simulink model "BatteryStoragePVPlantGFM"  (R2023a)
settings: Solver=FixedStepDiscrete  StartTime=0.0  StopTime=SimulationTime  RelTol=1e-3
PreLoadFcn:
  | run('BatteryStoragePVPlantGFMParameters')
undefined symbols (not defined in the file): Array, Base, battery, BatteryInverter, DiscIntNeverNeededParam, ee, Feeder, fRT, GFLBatteryController, GFMBatteryController, Grid, GridTransformer, Line, Load, Load2CB_final, Load2CB_initial, LVRT, maxSoC, maxVdc, minIrrad, minSoC, minVdc, Mpp, olTime, Panel, PVController, PVInverter, PVTransformer, Scenario, SM, SubTransmissionLine, Ts, VSMbase
libraries: ee_lib x51, nesl_utility x45, fl_lib x26, eeGeneralControl x18, simulink x12, eeTransforms x11, slpidlib x8, eePowerMeasurement x5, batteryecm_lib x2, eeTotalHarmonicDistorsion x2, spsLeadLagFilterLib x1, eeSmAC1C x1
(part 2 of 5)

== system BatteryStoragePVPlantGFM/Transmission Line/CB ==
  Circuit Breaker Step off3 : ee_lib/Switches & Breakers/Circuit Breaker (Three-Phase)  R_closed=0.001 Ohm  G_open=1e-4 1/Ohm  threshold=0.5 V  breaker_behavior=ee.enum.switches.breakerBehavior.zeroCrossingEnable
      settings: InternalSimscapePortConfiguration="{\"Bottom\":[],\"Left\":[{\"id\":\"vT\",\"label\":\"vT\",\"type\":\"input\"},{\"id\":\"N1\",\"label\":\"~1\",\"type\":\"foundation.electrical.three_phase\"}],\"Right\":[{\"id\":\"N2\",\"label\":\"~2\",\"type\":\"foundation.electrical.three_phase\"}],\"Top\":[]}"
  Constant : Constant  Value=0
  Simulink-PS Converter3 : nesl_utility/Simulink-PS Converter  PhysicalDomain=network_engine_domain  SubClassName=ps_input  LeftPortType=input  RightPortType=output  PseudoPeriodic=off  Frequencies=[]  NoiseDistribution=none  NoiseParameters=[]  Unit=1  AffineConversion=off  FilteringAndDerivatives=zero  SimscapeFilterOrder=1  InputFilterTimeConstant=0.001  UdotUserProvided=1
  Conn1 : PMIOPort  Side=Right
  Conn2 : PMIOPort  Port=2  Side=Left
  wires:
  Constant/1 -> Simulink-PS Converter3/1
  connections:
  Circuit Breaker Step off3/LConn2 -- Conn2/RConn1
  Circuit Breaker Step off3/LConn1 -- Simulink-PS Converter3/RConn1
  Circuit Breaker Step off3/RConn1 -- Conn1/RConn1

== system BatteryStoragePVPlantGFM/Transmission Line/CB5 ==
  Circuit Breaker Step off3 : ee_lib/Switches & Breakers/Circuit Breaker (Three-Phase)  R_closed=0.001 Ohm  G_open=1e-4 1/Ohm  threshold=0.5 V  breaker_behavior=ee.enum.switches.breakerBehavior.zeroCrossingEnable
      settings: InternalSimscapePortConfiguration="{\"Bottom\":[],\"Left\":[{\"id\":\"vT\",\"label\":\"vT\",\"type\":\"input\"},{\"id\":\"N1\",\"label\":\"~1\",\"type\":\"foundation.electrical.three_phase\"}],\"Right\":[{\"id\":\"N2\",\"label\":\"~2\",\"type\":\"foundation.electrical.three_phase\"}],\"Top\":[]}"
  Constant : Constant  Value=0
  Simulink-PS Converter3 : nesl_utility/Simulink-PS Converter  PhysicalDomain=network_engine_domain  SubClassName=ps_input  LeftPortType=input  RightPortType=output  PseudoPeriodic=off  Frequencies=[]  NoiseDistribution=none  NoiseParameters=[]  Unit=1  AffineConversion=off  FilteringAndDerivatives=zero  SimscapeFilterOrder=1  InputFilterTimeConstant=0.001  UdotUserProvided=1
  Conn1 : PMIOPort  Side=Right
  Conn2 : PMIOPort  Port=2  Side=Left
  wires:
  Constant/1 -> Simulink-PS Converter3/1
  connections:
  Circuit Breaker Step off3/LConn2 -- Conn2/RConn1
  Circuit Breaker Step off3/LConn1 -- Simulink-PS Converter3/RConn1
  Circuit Breaker Step off3/RConn1 -- Conn1/RConn1

== system BatteryStoragePVPlantGFM/BESS & PV PARK/100 MWp PV Park/Measurement1 ==
  u : Inport
  Lead-Lag (Discrete or Continuous) : eeGeneralControl/Lead-Lag (Discrete or Continuous)  T1=0  T2=PVController.t_sensor  B=inf  A=-inf  init_option=Inherited from block input  x0=0  Ts=Ts
      settings: LibrarySourceBlock=|
      | ee_sl_lib/General Control/Lead-Lag
      | (Discrete or Continuous)
  Out Bus Element : Outport  PortName=ipv1  Element=1
  wires:
  Lead-Lag (Discrete or Continuous)/1 -> Out Bus Element/1
  u/1 -> Lead-Lag (Discrete or Continuous)/1

== system BatteryStoragePVPlantGFM/BESS & PV PARK/100 MWp PV Park/Measurement2 ==
  u : Inport
  Lead-Lag (Discrete or Continuous) : eeGeneralControl/Lead-Lag (Discrete or Continuous)  T1=0  T2=PVController.t_sensor  B=inf  A=-inf  init_option=Inherited from block input  x0=0  Ts=Ts
      settings: LibrarySourceBlock=|
      | ee_sl_lib/General Control/Lead-Lag
      | (Discrete or Continuous)
  Out Bus Element : Outport  PortName=ipv1  Element=1
  wires:
  u/1 -> Lead-Lag (Discrete or Continuous)/1
  Lead-Lag (Discrete or Continuous)/1 -> Out Bus Element/1

== system BatteryStoragePVPlantGFM/BESS & PV PARK/100 MWp PV Park/PV Inverter A1 ==
  note: Voltage reference for the PV inverter
  Insolation : Inport
  In Bus Element : Inport  Port=2  PortName=Vbus
  In Bus Element2 : Inport  Port=3  PortName=LVRT
  In Bus Element1 : Inport  Port=4  PortName=ipv1
  Q_ref : Inport  Port=5
  PV & Inverter : Subsystem
  PV Controller : Subsystem
  abc : PMIOPort  Side=Right
  wires:
  Insolation/1 -> PV & Inverter/1(Solar insolation)
  [m] -> PV & Inverter/2(reference)
  In Bus Element2/1 -> PV Controller/3(LVRT)
  In Bus Element/1 -> PV Controller/4(Vbus)
  PV & Inverter/1(PV_plant1) -> PV Controller/1(PV_plant1)
  In Bus Element1/1 -> PV Controller/2(ipv1)
  PV Controller/1(m_abc) -> [m]
  Q_ref/1 -> PV Controller/5(Q_ref)
  connections:
  abc/RConn1 -- PV & Inverter/RConn1

== system BatteryStoragePVPlantGFM/BESS & PV PARK/100 MWp PV Park/PV Inverter A2 ==
  note: Voltage reference for the PV inverter
  Insolation : Inport
  In Bus Element : Inport  Port=2  PortName=Vbus
  In Bus Element2 : Inport  Port=3  PortName=LVRT
  In Bus Element1 : Inport  Port=4  PortName=ipv1
  Q_ref : Inport  Port=5
  PV & Inverter : Subsystem
  PV Controller : Subsystem
  abc : PMIOPort  Side=Right
  wires:
  Insolation/1 -> PV & Inverter/1(Solar insolation)
  [m] -> PV & Inverter/2(reference)
  In Bus Element2/1 -> PV Controller/3(LVRT)
  In Bus Element/1 -> PV Controller/4(Vbus)
  PV & Inverter/1(PV_plant1) -> PV Controller/1(PV_plant1)
  In Bus Element1/1 -> PV Controller/2(ipv1)
  PV Controller/1(m_abc) -> [m]
  Q_ref/1 -> PV Controller/5(Q_ref)
  connections:
  abc/RConn1 -- PV & Inverter/RConn1

== system BatteryStoragePVPlantGFM/BESS & PV PARK/60 MWhr Battery Energy Storage/Variant Subsystem ==
  Vbus : Inport
  LVRT : Inport  Port=2
  Grid Following Support : Subsystem  VariantControl=BESSGridSupporting
      mask Display: image('$imagefile'); % Use "Edit Image" on toolstrip to change.
  Grid Forming VSM : Subsystem  VariantControl=BESSVSMControl
      mask Display: image('$imagefile'); % Use "Edit Image" on toolstrip to change.
  GFL1 : PMIOPort  Side=Left
  Bat : Outport

== system BatteryStoragePVPlantGFM/BESS & PV PARK/PV Plant Controller /Logging Signals  ==
  Bus Element In1 : Inport  PortName=Measure  Element=P_total
  Bus Element In2 : Inport  PortName=Measure  Element=Q_total
  Bus Element In3 : Inport  PortName=Measure  Element=P_Bat
  Bus Element In4 : Inport  PortName=Measure  Element=Q_Bat
  Bus Element In5 : Inport  PortName=Measure  Element=P_PV
  Bus Element In6 : Inport  PortName=Measure  Element=Q_PV
  In Bus Element : Inport  Port=2  PortName=Vbus  Element=Vmag
  In Bus Element1 : Inport  Port=2  PortName=Vbus  Element=w
  In Bus Element2 : Inport  Port=2  PortName=Vbus  Element=Vabc
  In Bus Element3 : Inport  Port=2  PortName=Vbus  Element=Iabc
  In Bus Element4 : Inport  Port=3  PortName=Bat  Element=Iabc_bat
  Bus Creator : BusCreator  Inputs=11
  Output : Outport
  wires:
  Bus Creator/1 -> Output/1
  Bus Element In1/1 -> Bus Creator/1
  Bus Element In2/1 -> Bus Creator/2
  In Bus Element/1 -> Bus Creator/3
  In Bus Element1/1 -> Bus Creator/4
  In Bus Element2/1 -> Bus Creator/5
  In Bus Element3/1 -> Bus Creator/6
  Bus Element In3/1 -> Bus Creator/7
  Bus Element In4/1 -> Bus Creator/8
  Bus Element In5/1 -> Bus Creator/9
  Bus Element In6/1 -> Bus Creator/10
  In Bus Element4/1 -> Bus Creator/11

== system BatteryStoragePVPlantGFM/BESS & PV PARK/PV Plant Controller /Power Measurements ==
  In Bus Element10 : Inport  PortName=Vbus  Element=Vabc
  In Bus Element2 : Inport  PortName=Vbus  Element=Vabc
  In Bus Element15 : Inport  PortName=Vbus  Element=Iabc
  In Bus Element3 : Inport  Port=2  PortName=Bat  Element=Iabc_bat
  In Bus Element1 : Inport  Port=2  PortName=Bat  Element=Vabc_bat
  ipv : Inport  Port=3
  Gain{,3..4,7} (4 alike) : Gain  Gain=(2/3)*Base.MVA_base_new
  Gain1 : Gain  Gain=1%(2/3)*Base.MVA_base_new
  Gain2 : Gain  Gain=1%(2/3)*Base.MVA_base_new
  Power Measurement (Three-Phase) : eePowerMeasurement/Power Measurement (Three-Phase)  LabelModeActiveChoice=Discrete  F=60  K=[1]  Seq=Positive  Ts=Ts
  Power Measurement (Three-Phase)1 : eePowerMeasurement/Power Measurement (Three-Phase)  LabelModeActiveChoice=Discrete  F=60  K=[1]  Seq=Positive  Ts=Ts
  Power Measurement (Three-Phase)2 : eePowerMeasurement/Power Measurement (Three-Phase)  LabelModeActiveChoice=Discrete  F=60  K=[1]  Seq=Positive  Ts=Ts
  Out Bus Element9 : Outport  PortName=Measure  Element=P_total
  Out Bus Element10 : Outport  PortName=Measure  Element=Q_total
  Out Bus Element1 : Outport  PortName=Measure  Element=P_Bat
  Out Bus Element2 : Outport  PortName=Measure  Element=Q_Bat
  Out Bus Element3 : Outport  PortName=Measure  Element=P_PV
  Out Bus Element4 : Outport  PortName=Measure  Element=Q_PV
  wires:
  Gain1/1 -> Out Bus Element1/1
  Gain/1 -> Out Bus Element9/1
  Gain7/1 -> Out Bus Element10/1
  In Bus Element2/1 -> Power Measurement (Three-Phase)2/1
  Gain4/1 -> Out Bus Element4/1
  Power Measurement (Three-Phase)2/2 -> Gain4/1
  Gain3/1 -> Out Bus Element3/1
  Power Measurement (Three-Phase)/2 -> Gain7/1
  Power Measurement (Three-Phase)1/1 -> Gain1/1
  Power Measurement (Three-Phase)2/1 -> Gain3/1
  Power Measurement (Three-Phase)/1 -> Gain/1
  Power Measurement (Three-Phase)1/2 -> Gain2/1
  Gain2/1 -> Out Bus Element2/1
  In Bus Element1/1 -> Power Measurement (Three-Phase)1/1
  In Bus Element3/1 -> Power Measurement (Three-Phase)1/2
  In Bus Element10/1 -> Power Measurement (Three-Phase)/1
  In Bus Element15/1 -> Power Measurement (Three-Phase)/2
  ipv/1 -> Power Measurement (Three-Phase)2/2

== system BatteryStoragePVPlantGFM/BESS & PV PARK/PV Plant Controller /Voltage VAR Control & LVRT, FRT ==
  In Bus Element : Inport  PortName=Vbus  Element=Vmag
  In Bus Element1 : Inport  PortName=Vbus  Element=w
  Data Type Conversion : DataTypeConversion  RndMeth=Nearest  SaturateOnIntegerOverflow=off
  Frequency RideThrough : Subsystem
  LVRT Characterstics : Subsystem
  OR : Logic  Operator=OR  IconShape=distinctive  AllPortsSameDT=off  OutDataTypeStr=boolean
  Unit Delay : UnitDelay  SampleTime=-1  HasFrameUpgradeWarning=on
  V_ref : Constant  Value=PVController.V_ref  SampleTime=Ts
  Voltage Control : Subsystem
  Out Bus Element : Outport  PortName=LVRT  Element=breaker
  Out Bus Element1 : Outport  PortName=LVRT  Element=iq
  Q_ref : Outport  Port=2
  wires:
  In Bus Element/1 -> LVRT Characterstics/1(Vmag), Voltage Control/1(In1)
  LVRT Characterstics/2(iq) -> Out Bus Element1/1
  V_ref/1 -> Voltage Control/2(In2)
  Voltage Control/1(Out1) -> Q_ref/1
  OR/1 -> Data Type Conversion/1
  LVRT Characterstics/1(Trip Signal) -> OR/1
  In Bus Element1/1 -> Frequency RideThrough/1(f)
  Data Type Conversion/1 -> Unit Delay/1
  Frequency RideThrough/1(Trip  Signal) -> OR/2
  Unit Delay/1 -> Out Bus Element/1

== system BatteryStoragePVPlantGFM/Conventional Source/Variant Subsystem/Frequency Controlled Source ==
  Grid : Inport
  Electrical Reference9 : fl_lib/Electrical/Electrical Elements/Electrical Reference
  Frequency Control : Subsystem
  P_ref : Constant  Value=Grid.Pref
  Programmable Voltage Source (Three-Phase) : ee_lib/Sources/Programmable Voltage Source (Three-Phase)  magnitude_type=ee.enum.timechanging.constant  vline_rms=Grid.voltage V  magn_ramp=1 V/s  magn_step=1 V  magn_modu_magn=1 V  magn_modu_freq=1 Hz  magn_t1=1 s  magn_t2=2 s  frequency_type=ee.enum.timechanging.external  freq=60 Hz  freq_ramp=1 Hz/s  freq_step=1 Hz  freq_modu_magn=1 Hz  freq_modu_freq=1 Hz  freq_t1=1 s  freq_t2=2 s  phase_type=ee.enum.timechanging.constant  shift=0 deg  phase_ramp=1 deg/s  phase_step=1 deg  phase_modu_magn=1 deg  phase_modu_freq=1 Hz  phase_t1=1 s  phase_t2=2 s  impedance_option=4  SShortCircuit=1e6 A*V  XR=15  R=Grid.Rs Ohm  L=Grid.Ls mH  G_parasitic=1e-6 1/Ohm  harmonic_option=0  harmonic_orders=[5, 7, 11, 13]  harmonic_ratios=[.1, .1, .1, .1]  harmonic_shifts=[0, 0, 0, 0] deg  harmonic_sequences=[1, 1, 1, 1]  harmonic_t1=-inf s  harmonic_t2=inf s  I_specify=off  I_priority=None  I=[0, 0, 0] A  I_nominal_specify=off  I_nominal_unit=A  I_nominal_value=1  V_specify=off  V_priority=None  V=[0, 0, 0] V  V_nominal_specify=off  V_nominal_unit=V  V_nominal_value=1
      settings: InternalSimscapePortConfiguration="{\"Bottom\":[],\"Left\":[{\"id\":\"ext_freq\",\"label\":\"F\",\"type\":\"input\"},{\"id\":\"n\",\"label\":\"n\",\"type\":\"foundation.electrical.electrical\"}],\"Right\":[{\"id\":\"N\",\"label\":\"~\",\"type\":\"foundation.electrical.three_phase\"}],\"Top\":[]}"
  Simulink-PS Converter : nesl_utility/Simulink-PS Converter  PhysicalDomain=network_engine_domain  SubClassName=ps_input  LeftPortType=input  RightPortType=output  PseudoPeriodic=off  Frequencies=[]  NoiseDistribution=none  NoiseParameters=[]  Unit=1  AffineConversion=off  FilteringAndDerivatives=provide  SimscapeFilterOrder=1  InputFilterTimeConstant=0.001  UdotUserProvided=0
  abc : PMIOPort  Side=Right
  Connection Port1 : PMIOPort  Port=2  Side=Left
  wires:
  Frequency Control/1(Frequency) -> Simulink-PS Converter/1
  Grid/1 -> Frequency Control/2(Grid)
  P_ref/1 -> Frequency Control/1(Pref)
  connections:
  Electrical Reference9/LConn1 -- Connection Port1/RConn1 -- Programmable Voltage Source (Three-Phase)/LConn2
  Simulink-PS Converter/RConn1 -- Programmable Voltage Source (Three-Phase)/LConn1
  abc/RConn1 -- Programmable Voltage Source (Three-Phase)/RConn1

== system BatteryStoragePVPlantGFM/Conventional Source/Variant Subsystem/Synchronous Machine ==
  " Load" : ee_lib/Passive/RLC Assemblies/Wye-Connected Load  parameterization=ee.enum.rlc.parameterization.ratedpower  component_structure=ee.enum.rlc.structure.R  component_structure_PQ=ee.enum.rlc.structure.ParallelRL  R=1 Ohm  L=1e-3 H  C=1e-6 F  VRated=Grid.voltage V  FRated=Grid.frequency Hz  P=SM.P_load W  Qpos=SM.Q_load A*V  Qneg=-1e2 A*V  R_parasitic=0 Ohm  G_parasitic=0 1/Ohm  R_parasitic_PQ=0 Ohm  G_parasitic_PQ=0 1/Ohm  Vmag0=4.16e3 V  Vang0=0 deg  Freq0=60 Hz  IL_specify=off  IL_priority=High  IL=[0, 0, 0] A  IL_nominal_specify=off  IL_nominal_unit=A  IL_nominal_value=1  VC_specify=off  VC_priority=High  VC=[0, 0, 0] V  VC_nominal_specify=off  VC_nominal_unit=V  VC_nominal_value=1
  230/24 kV : ee_lib/Passive/Transformers/Two-Winding Transformer (Three-Phase)  SRated=500e6 V*A  FRated=60 Hz  Winding1Connection=ee.enum.windingconnection.delta1  VRated1=GridTransformer.hv V  Winding2Connection=ee.enum.windingconnection.delta11  VRated2=24e3 V  CoreType=ee.enum.coretype.fivelimb  pu_Rw1=GridTransformer.winding_resistance/2  pu_Rw2=GridTransformer.winding_resistance/2  leakage_reactance_option=ee.enum.transformer_leakage.include  pu_Xl1=GridTransformer.winding_lekage_reactance/2  pu_Xl2=GridTransformer.winding_lekage_reactance/2  magnetizing_resistance_option=ee.enum.transformer_magnetizingResistance.exclude  pu_Rm=500  magnetizing_reactance_option=ee.enum.transformer_magnetizingReactance.include  saturation_option=ee.enum.transformer_saturation.exclude  pu_Xm=500  current_data=[0, .002, 1, 2]  magnetic_flux_data=[0, 1.2, 1.5, 1.51]  pu_X0=0.0586/2  i1_specify=off  i1_priority=None  i1=[ 0 0 0 ] A  i1_nominal_specify=off  i1_nominal_unit=A  i1_nominal_value=1  i2_specify=off  i2_priority=None  i2=[ 0 0 0 ] A  i2_nominal_specify=off  i2_nominal_unit=A  i2_nominal_value=1  phi_specify=off  phi_priority=None  phi=[ 0 0 0 ]  phi_nominal_specify=off  phi_nominal_unit=1  phi_nominal_value=1  power_dissipated_specify=off  power_dissipated_priority=None  power_dissipated=0 W  power_dissipated_nominal_specify=off  power_dissipated_nominal_unit=W  power_dissipated_nominal_value=1
      settings: InternalSimscapePortConfiguration="{\"Bottom\":[],\"Left\":[{\"id\":\"N1\",\"label\":\"~1\",\"type\":\"foundation.electrical.three_phase\"}],\"Right\":[{\"id\":\"N2\",\"label\":\"~2\",\"type\":\"foundation.electrical.three_phase\"}],\"Top\":[]}"
  AVR and Exciter : Subsystem
  CB4 : Subsystem
      settings: PortSchema="{\"entries\":[{\"content\":{\"sides\":[{\"content\":{\"connectorIds\":[\"LConn1\"]},\"type\":\"ConnectorPlacement.EquallySpacedRectSide\",\"uuid\":\"24022911-97b6-486c-a625-f0780a134feb\"},{\"content\":{\"connectorIds\":[],\"side\":\"RIGHT\"},\"type\":\"ConnectorPlacement.EquallySpacedRectSide\",\"uuid\":\"1242aa8b-343b-4af2-8b96-dfa58505a53d\"},{\"content\":{\"connectorIds\":[],\"side\":\"TOP\"},\"type\":\"ConnectorPlacement.EquallySpacedRectSide\",\"uuid\":\"e73be2e9-5300-480f-914f-665ff518f6ad\"},{\"content\":{\"connectorIds\":[\"RConn1\"],\"side\":\"BOTTOM\"},\"type\":\"ConnectorPlacement.EquallySpacedRectSide\",\"uuid\":\"6525202c-c4e7-4c96-9421-427b801d0594\"}]},\"type\":\"ConnectorPlacement.EquallySpacedConnector\",\"uuid\":\"b455682c-e951-4ef6-bff8-cd3f50b315f1\"}],\"packageUris\":[\"http://schema.mathworks.com/mf0/Connector/R2020b\"],\"version\":\"1.0\"}"
      mask Display: image('$imagefile'); % Use "Edit Image" on toolstrip to change.
  Current and Voltage Sensor (Three-Phase)1 : ee_lib/Sensors & Transducers/Current and Voltage Sensor (Three-Phase)  vMeasurementType=ee.enum.vmeasurement.ll  outputUnit=ee.enum.unit.pu  SRated=100e6 A*V  VRated=4.16e3 V  I_specify=off  I_priority=None  I=[0, 0, 0] A  I_nominal_specify=off  I_nominal_unit=A  I_nominal_value=1  V_specify=off  V_priority=None  V=[0, 0, 0] V  V_nominal_specify=off  V_nominal_unit=V  V_nominal_value=1
      settings: InternalSimscapePortConfiguration="{\"Bottom\":[],\"Left\":[{\"id\":\"N1\",\"label\":\"~1\",\"type\":\"foundation.electrical.three_phase\"}],\"Right\":[{\"id\":\"V_output\",\"label\":\"V\",\"type\":\"output\"},{\"id\":\"I_output\",\"label\":\"I\",\"type\":\"output\"},{\"id\":\"N2\",\"label\":\"~2\",\"type\":\"foundation.electrical.three_phase\"}],\"Top\":[]}"
  Electrical Reference1 : fl_lib/Electrical/Electrical Elements/Electrical Reference
  Electrical Reference2 : fl_lib/Electrical/Electrical Elements/Electrical Reference
  "Governor and Prime Mover " : Subsystem  mask(Governor and Prime Mover){pu_speed_reference=SM.speed_reference, droop_percentage=SM.droop_p, pu_load_reference_setpoint=SM.load_reference_set_point, T_G=SM.governor_time_constant, T_CH=SM.time_constsnt_steamchest, base_torque=SM.Base_Torque_SM, pu_torque0=SM.initial_torque}
      mask prompts: pu_speed_reference "Speed reference, (pu)"; droop_percentage "Percentage droop, (%)"; pu_load_reference_setpoint "Load reference setpoint, (pu)"; T_G "Time constant of governor, (s)"; T_CH "Time constant of main inlet volumes and steam chest, (s)"; base_torque "Base torque, (N*m)"; pu_torque0 "Initial torque, (pu)"
      mask help:
      | Implements a synchronous machine governor and prime mover. The prime mover is a non-reheat steam turbine.
      |
      | The input to the block is a per-unit synchronous machine measurement vector.
      |
      | R and C are mechanical rotational ports.
  Machine Inertia : ee_lib/Electromechanical/Mechanical/Machine Inertia  SRated=SM.MVA V*A  FRated=Grid.frequency Hz  nPolePairs=SM.polepairs  inertia_option=2  J=27548 kg*m^2  H=SM.inertia s  damper_option=2  D=39.0509 N*m/(rad/s)  pu_D=SM.damping  initialization_option=2  fMechanical0=60 Hz  fElectrical0=Grid.frequency Hz
      settings: InternalSimscapePortConfiguration="{\"Bottom\":[],\"Left\":[{\"id\":\"R\",\"label\":\"R\",\"type\":\"foundation.mechanical.rotational.rotational\"}],\"Right\":[],\"Top\":[]}"
  PS-Simulink Converter : nesl_utility/PS-Simulink Converter  PhysicalDomain=network_engine_domain  SubClassName=ps_output  LeftPortType=input  RightPortType=output  PseudoPeriodic=off  Frequencies=[]  VectorFormat=inherit  Unit=inherit  AffineConversion=off
  PS-Simulink Converter1 : nesl_utility/PS-Simulink Converter  PhysicalDomain=network_engine_domain  SubClassName=ps_output  LeftPortType=input  RightPortType=output  PseudoPeriodic=off  Frequencies=[]  VectorFormat=inherit  Unit=inherit  AffineConversion=off
  SM Round Rotor (standard) : ee_lib/Electromechanical/Synchronous/Synchronous Machine Round Rotor  port_option=ee.enum.threePhasePort.composite  SRated=SM.MVA V*A  VRated=SM.Voltage V  FRated=Grid.frequency Hz  nPolePairs=SM.polepairs  param_option=ee.enum.sm.parameterization.standard  fieldCircuitParameterization_option=2  baseEfd=92.95 V  baseIfd=SM.field_current A  zero_sequence=ee.enum.park.zerosequence.include  axes_param=ee.enum.rotorangle.qaxis  Ladu=1.66  Laqu=1.61  L0=0.15  Ll=0.15  Ra=SM.stator_resistance  Lfd=0.165  Rfd=0.0006  L1d=0.1713  R1d=0.0284  L1q=0.7252  R1q=0.00619  L2q=0.125  R2q=0.02368  Xl=SM.lekage_reactance  Xd=SM.xd  Xq=SM.xq  X0=0.15  Xdd=SM.xd_  Xqd=SM.xq_  Xddd=SM.xd_dash  Xqdd=SM.xq_dash  d_option=1  Td0d=SM.Tdo_ s  Tdd=1.3260 s  Td0dd=SM.Tdo_dash s  Tddd=0.0230 s  q_option=1  Tq0d=SM.Tqo_ s  Tqd=0.3693 s  Tq0dd=SM.Tqo_dash s  Tqdd=0.0269 s  saturation_option=0  saturation_ifd=[0.00, 0.48, 0.76, 1.38, 1.79]  saturation_Vag=[0.00, 0.80, 1.08, 1.31, 1.40]  initialization_option=2  source_type=ee.enum.sm.load_flow_source_type.Swing  Vmag0=SM.Voltage V  Vang0=0 deg  Pt0=SM.initial_Pe V*A  Qt0=SM.initial_Qe V*A  minimum_pu=0.95  phase_search_range=[-inf, inf] deg  gmin=1e-6 S  connection_option=int32(ee.enum.Connection.wye)  num_q_dampers=2  rotor_offset=-pi / 2 rad  pu_psid_specify=on  pu_psid_priority=High  pu_psid=0  pu_psid_nominal_specify=off  pu_psid_nominal_unit=1  pu_psid_nominal_value=1  pu_psiq_specify=on  pu_psiq_priority=High  pu_psiq=0  pu_psiq_nominal_specify=off  pu_psiq_nominal_unit=1  pu_psiq_nominal_value=1  pu_psifd_specify=on  pu_psifd_priority=High  pu_psifd=0  pu_psifd_nominal_specify=off  pu_psifd_nominal_unit=1  pu_psifd_nominal_value=1  pu_psi1d_specify=on  pu_psi1d_priority=High  pu_psi1d=0  pu_psi1d_nominal_specify=off  pu_psi1d_nominal_unit=1  pu_psi1d_nominal_value=1  pu_psi1q_specify=on  pu_psi1q_priority=High  pu_psi1q=0  pu_psi1q_nominal_specify=off  pu_psi1q_nominal_unit=1  pu_psi1q_nominal_value=1  pu_psi2q_specify=on  pu_psi2q_priority=High  pu_psi2q=0  pu_psi2q_nominal_specify=off  pu_psi2q_nominal_unit=1  pu_psi2q_nominal_value=1  angular_position_diff_specify=on  angular_position_diff_priority=High  angular_position_diff=0 deg  angular_position_diff_nominal_specify=off  angular_position_diff_nominal_unit=deg  angular_position_diff_nominal_value=1  Tmeas=298.15 K  alpha=3.93e-3 1/K  stator_thermal_mass=100 J/K  rotor_thermal_mass=200 J/K  temperatureA_specify=off  temperatureA_priority=High  temperatureA=25 degC  temperatureA_nominal_specify=off  temperatureA_nominal_unit=degC  temperatureA_nominal_value=1  temperatureB_specify=off  temperatureB_priority=High  temperatureB=25 degC  temperatureB_nominal_specify=off  temperatureB_nominal_unit=degC  temperatureB_nominal_value=1  temperatureC_specify=off  temperatureC_priority=High  temperatureC=25 degC  temperatureC_nominal_specify=off  temperatureC_nominal_unit=degC  temperatureC_nominal_value=1  temperatureR_specify=off  temperatureR_priority=High  temperatureR=25 degC  temperatureR_nominal_specify=off  temperatureR_nominal_unit=degC  temperatureR_nominal_value=1
      settings: InternalSimscapePortConfiguration="{\"Bottom\":[],\"Left\":[{\"id\":\"fd_p\",\"label\":\"fd+\",\"type\":\"foundation.electrical.electrical\"},{\"id\":\"fd_n\",\"label\":\"fd-\",\"type\":\"foundation.electrical.electrical\"},{\"id\":\"R\",\"label\":\"R\",\"type\":\"foundation.mechanical.rotational.rotational\"},{\"id\":\"C\",\"label\":\"C\",\"type\":\"foundation.mechanical.rotational.rotational\"}],\"Right\":[{\"id\":\"pu_output\",\"label\":\"pu\",\"type\":\"output\"},{\"id\":\"N\",\"label\":\"~\",\"type\":\"foundation.electrical.three_phase\"},{\"id\":\"n\",\"label\":\"n\",\"type\":\"foundation.electrical.electrical\"}],\"Top\":[]}"
  Terminator : Terminator
  Terminator1 : Terminator
  abc : PMIOPort  Side=Right
  Connection Port1 : PMIOPort  Port=2  Side=Left
  wires:
  PS-Simulink Converter/1 -> Terminator/1
  PS-Simulink Converter1/1 -> Terminator1/1
  connections:
  " Load"/LConn1 -- abc/RConn1 -- 230/24 kV/LConn1
  "Governor and Prime Mover "/LConn1 -- AVR and Exciter/LConn1 -- Connection Port1/RConn1 -- SM Round Rotor (standard)/RConn1
  SM Round Rotor (standard)/LConn3 -- Machine Inertia/LConn1 -- "Governor and Prime Mover "/RConn1
  SM Round Rotor (standard)/LConn4 -- "Governor and Prime Mover "/RConn2
  Current and Voltage Sensor (Three-Phase)1/RConn1 -- PS-Simulink Converter/LConn1
  SM Round Rotor (standard)/LConn1 -- AVR and Exciter/RConn1
  CB4/LConn1 -- Current and Voltage Sensor (Three-Phase)1/LConn1
  Electrical Reference1/LConn1 -- " Load"/RConn1
  SM Round Rotor (standard)/LConn2 -- AVR and Exciter/RConn2
  Current and Voltage Sensor (Three-Phase)1/RConn3 -- 230/24 kV/RConn1
  PS-Simulink Converter1/LConn1 -- Current and Voltage Sensor (Three-Phase)1/RConn2
  CB4/RConn1 -- SM Round Rotor (standard)/RConn2
  Electrical Reference2/LConn1 -- SM Round Rotor (standard)/RConn3

== system BatteryStoragePVPlantGFM/Measurements & PLL/PLL & Measurements/Measurement1 ==
  u : Inport
  Lead-Lag (Discrete or Continuous) : eeGeneralControl/Lead-Lag (Discrete or Continuous)  T1=0  T2=PVController.t_sensor  B=inf  A=-inf  init_option=Inherited from block input  x0=0  Ts=Ts
      settings: LibrarySourceBlock=|
      | ee_sl_lib/General Control/Lead-Lag
      | (Discrete or Continuous)
  Vg : Outport
  wires:
  Lead-Lag (Discrete or Continuous)/1 -> Vg/1
  u/1 -> Lead-Lag (Discrete or Continuous)/1

== system BatteryStoragePVPlantGFM/Measurements & PLL/PLL & Measurements/Measurement2 ==
  u : Inport
  Lead-Lag (Discrete or Continuous) : eeGeneralControl/Lead-Lag (Discrete or Continuous)  T1=0  T2=PVController.t_sensor  B=inf  A=-inf  init_option=Inherited from block input  x0=0  Ts=Ts
      settings: LibrarySourceBlock=|
      | ee_sl_lib/General Control/Lead-Lag
      | (Discrete or Continuous)
  Vg : Outport
  wires:
  Lead-Lag (Discrete or Continuous)/1 -> Vg/1
  u/1 -> Lead-Lag (Discrete or Continuous)/1

== system BatteryStoragePVPlantGFM/Measurements & PLL/PLL & Measurements/Subsystem ==
  Vabc : Inport
  Iabc : Inport  Port=2
  Demux : Demux  Outputs=3
  Demux1 : Demux  Outputs=3
  Park Transform : eeTransforms/Park Transform  AxisAlignment=Q-axis  PowerInvariant=off
  Park Transform1 : eeTransforms/Park Transform  AxisAlignment=Q-axis  PowerInvariant=off
  "Sinusoidal Measurement (PLL, Three-Phase)" : eeSinusoidalMeasurementV2/Sinusoidal Measurement (PLL, Three-Phase)  Kp_LF=PLL.Kp_pll  Ki_LF=PLL.Ki_pll  F0=Grid.frequency  Theta0=0  Ts=Ts
  Terminator : Terminator
  Terminator1 : Terminator
  mag : Outport
  freq : Outport  Port=2
  angle : Outport  Port=3
  Vd : Outport  Port=4
  Vq : Outport  Port=5
  Id1 : Outport  Port=6
  Iq1 : Outport  Port=7
  wires:
  Demux/3 -> Terminator/1
  Vabc/1 -> Park Transform/1, "Sinusoidal Measurement (PLL, Three-Phase)"/1
  Park Transform/1 -> Demux/1
  Demux/1 -> Vd/1
  Demux/2 -> Vq/1
  "Sinusoidal Measurement (PLL, Three-Phase)"/2 -> angle/1, Park Transform1/2, Park Transform/2
  "Sinusoidal Measurement (PLL, Three-Phase)"/1 -> freq/1
  "Sinusoidal Measurement (PLL, Three-Phase)"/3 -> mag/1
  Park Transform1/1 -> Demux1/1
  Demux1/1 -> Id1/1
  Demux1/2 -> Iq1/1
  Demux1/3 -> Terminator1/1
  Iabc/1 -> Park Transform1/1

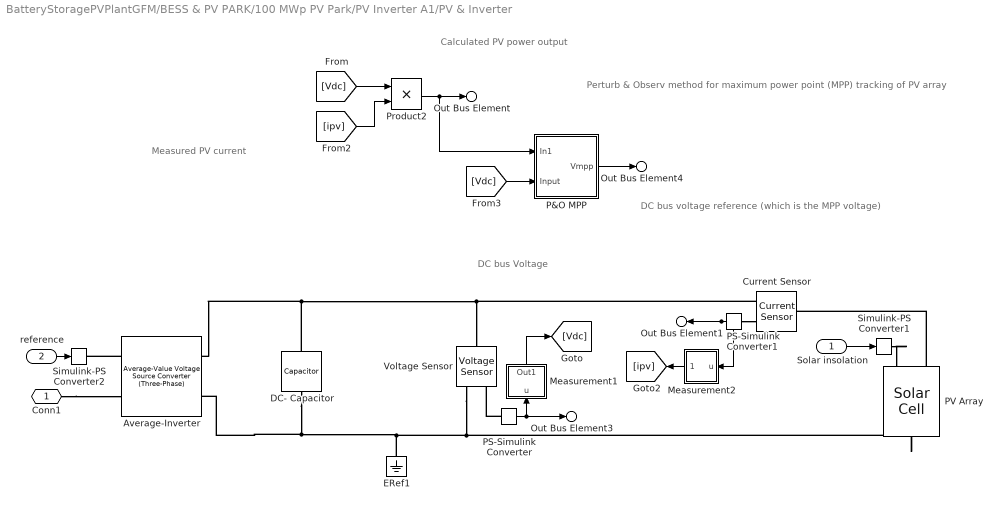
== system BatteryStoragePVPlantGFM/BESS & PV PARK/100 MWp PV Park/PV Inverter A1/PV & Inverter ==
  note: DC bus Voltage
  note: DC bus voltage reference (which is the MPP voltage)
  note: Perturb & Observ method for maximum power point (MPP) tracking of PV array
  note: Measured PV current
  note: Calculated PV power output
  Solar insolation : Inport
  reference : Inport  Port=2
  Average-Inverter : ee_lib/Semiconductors & Converters/Converters/Average-Value Voltage Source Converter (Three-Phase)  port_option=ee.enum.threePhasePort.composite  frequency_option=ee.enum.converters.frequency.variable  FRated=60 Hz  losses_parameterization=ee.enum.converters.losses.fixed  Pfixed=1 W  ks=0.01  kc1=1.7 V  kc2=0.01 Ohm  Ploss_vect=[100, 800, 1870, 3250, 4900] W  Irms_vect=[10, 100, 200, 300, 400] A  Vdc_nom=300 V  thermal_mass=30000 J/K  temperature_specify=off  temperature_priority=High  temperature=298.15 K  temperature_nominal_specify=off  temperature_nominal_unit=K  temperature_nominal_value=1
      settings: InternalSimscapePortConfiguration="{\"Bottom\":[],\"Left\":[{\"id\":\"ModWave\",\"label\":\"ModWave\",\"type\":\"input\"},{\"id\":\"N\",\"label\":\"~\",\"type\":\"foundation.electrical.three_phase\"}],\"Right\":[{\"id\":\"p\",\"label\":\"+\",\"type\":\"foundation.electrical.electrical\"},{\"id\":\"n\",\"label\":\"-\",\"type\":\"foundation.electrical.electrical\"}],\"Top\":[]}"
  Current Sensor : fl_lib/Electrical/Electrical Sensors/Current Sensor
  DC- Capacitor : fl_lib/Electrical/Electrical Elements/Capacitor  c=PVInverter.C F  r=1e-6 Ohm  g=0 1/Ohm  i_specify=off  i_priority=None  i=0 A  i_nominal_specify=off  i_nominal_unit=A  i_nominal_value=1  v_specify=off  v_priority=None  v=6560*.5 V  v_nominal_specify=off  v_nominal_unit=V  v_nominal_value=1  vc_specify=on  vc_priority=None  vc=PVInverter.Vdc V  vc_nominal_specify=off  vc_nominal_unit=V  vc_nominal_value=1
  ERef1 : fl_lib/Electrical/Electrical Elements/Electrical Reference
  Measurement1 : Subsystem
  Measurement2 : Subsystem
  P&O MPP : Subsystem
  PS-Simulink Converter : nesl_utility/PS-Simulink Converter  PhysicalDomain=network_engine_domain  SubClassName=ps_output  LeftPortType=input  RightPortType=output  PseudoPeriodic=off  Frequencies=[]  VectorFormat=inherit  Unit=inherit  AffineConversion=off
  PS-Simulink Converter1 : nesl_utility/PS-Simulink Converter  PhysicalDomain=network_engine_domain  SubClassName=ps_output  LeftPortType=input  RightPortType=output  PseudoPeriodic=off  Frequencies=[]  VectorFormat=inherit  Unit=inherit  AffineConversion=off
  PV Array : ee_lib/Sources/Solar Cell  prm=3  Isc=3.8 A  Voc=0.586 V  Is=SolarCell.diode_saturation_current A  Is2=0 A  Iph=SolarCell.solar_generated_current_AM A  Ir0=1000 W/m^2  ec=SolarCell.quality_factor_i  N2=SolarCell.quality_factor_j  Rs=SolarCell.series_resistance Ohm  Rp=SolarCell.parallel_resistance Ohm  N_series=Panel.n_series_cell_panel*Array.n_series_panels_per_string  N_parallel=Panel.n_parallel_strings_panel*Array.n_parallel_strings  TIPH1=SolarCell.temp_cofficient 1/K  EG=SolarCell.Eg eV  TXIS1=SolarCell.temperature_exponent_Is1  TXIS2=SolarCell.temperature_exponent_Is2  TRS1=SolarCell.temperature_exponent_Rs  TRP1=SolarCell.temperature_exponent_Rp  Tmeas=SolarCell.measurement_temperature degC  TFIXED=SolarCell.device_temperature degC  thermal_mass=100 J/K  initial_temperature=25 degC
  Product2 : Product
  Simulink-PS Converter1 : nesl_utility/Simulink-PS Converter  PhysicalDomain=network_engine_domain  SubClassName=ps_input  LeftPortType=input  RightPortType=output  PseudoPeriodic=off  Frequencies=[]  NoiseDistribution=none  NoiseParameters=[]  Unit=1  AffineConversion=off  FilteringAndDerivatives=provide  SimscapeFilterOrder=1  InputFilterTimeConstant=0.001  UdotUserProvided=0
  Simulink-PS Converter2 : nesl_utility/Simulink-PS Converter  PhysicalDomain=network_engine_domain  SubClassName=ps_input  LeftPortType=input  RightPortType=output  PseudoPeriodic=off  Frequencies=[]  NoiseDistribution=none  NoiseParameters=[]  Unit=1  AffineConversion=off  FilteringAndDerivatives=provide  SimscapeFilterOrder=1  InputFilterTimeConstant=0.001  UdotUserProvided=0
  Voltage Sensor : fl_lib/Electrical/Electrical Sensors/Voltage Sensor
  Conn1 : PMIOPort  Side=Right
  Out Bus Element4 : Outport  PortName=PV_plant1  Element=Vdc_ref
  Out Bus Element : Outport  PortName=PV_plant1  Element=Pref1
  Out Bus Element3 : Outport  PortName=PV_plant1  Element=Vdc_measured
  Out Bus Element1 : Outport  PortName=PV_plant1  Element=ipv
  wires:
  PS-Simulink Converter1/1 -> Measurement2/1(u), Out Bus Element1/1
  Solar insolation/1 -> Simulink-PS Converter1/1
  [ipv] -> Product2/2
  PS-Simulink Converter/1 -> Measurement1/1(u), Out Bus Element3/1
  [Vdc] -> Product2/1
  reference/1 -> Simulink-PS Converter2/1
  Product2/1 -> P&O MPP/1(In1), Out Bus Element/1
  P&O MPP/1(Vmpp) -> Out Bus Element4/1
  [Vdc] -> P&O MPP/2(Input)
  Measurement1/1(Out1) -> [Vdc]
  Measurement2/1(Out1) -> [ipv]
  connections:
  PS-Simulink Converter/LConn1 -- Voltage Sensor/RConn1
  DC- Capacitor/LConn1 -- Current Sensor/RConn2 -- Voltage Sensor/LConn1 -- Average-Inverter/RConn1
  Voltage Sensor/RConn2 -- DC- Capacitor/RConn1 -- Average-Inverter/RConn2 -- ERef1/LConn1 -- PV Array/RConn1
  Average-Inverter/LConn1 -- Simulink-PS Converter2/RConn1
  PV Array/LConn2 -- Current Sensor/LConn1
  Conn1/RConn1 -- Average-Inverter/LConn2
  PS-Simulink Converter1/LConn1 -- Current Sensor/RConn1
  Simulink-PS Converter1/RConn1 -- PV Array/LConn1

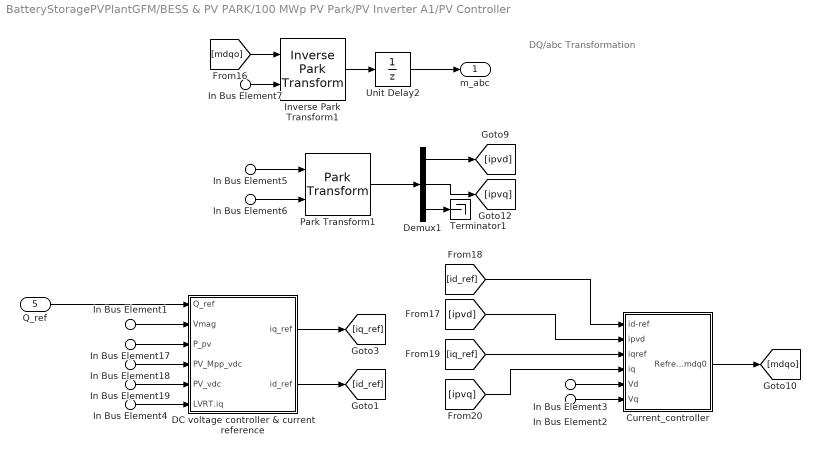
== system BatteryStoragePVPlantGFM/BESS & PV PARK/100 MWp PV Park/PV Inverter A1/PV Controller ==
  note: DQ/abc Transformation
  In Bus Element17 : Inport  PortName=PV_plant1  Element=Pref1
  In Bus Element18 : Inport  PortName=PV_plant1  Element=Vdc_measured
  In Bus Element19 : Inport  PortName=PV_plant1  Element=Vdc_ref
  In Bus Element5 : Inport  Port=2  PortName=ipv1  Element=1
  In Bus Element4 : Inport  Port=3  PortName=LVRT
  In Bus Element3 : Inport  Port=4  PortName=Vbus  Element=Vd
  In Bus Element1 : Inport  Port=4  PortName=Vbus  Element=Vd
  In Bus Element2 : Inport  Port=4  PortName=Vbus  Element=Vq
  In Bus Element6 : Inport  Port=4  PortName=Vbus  Element=Theta
  In Bus Element7 : Inport  Port=4  PortName=Vbus  Element=Theta
  Q_ref : Inport  Port=5
  Current_controller : Subsystem
  DC voltage controller & current reference : Subsystem
  Demux1 : Demux  Outputs=3
  Inverse Park Transform1 : eeTransforms/Inverse Park Transform  AxisAlignment=Q-axis  PowerInvariant=off
  Park Transform1 : eeTransforms/Park Transform  AxisAlignment=Q-axis  PowerInvariant=off
  Terminator1 : Terminator
  Unit Delay2 : UnitDelay  SampleTime=Ts  HasFrameUpgradeWarning=on
  m_abc : Outport
  wires:
  In Bus Element2/1 -> Current_controller/6(Vq)
  Current_controller/1(Refrence_mdq0) -> [mdqo]
  Inverse Park Transform1/1 -> Unit Delay2/1
  Demux1/2 -> [ipvq]
  Unit Delay2/1 -> m_abc/1
  Demux1/1 -> [ipvd]
  Demux1/3 -> Terminator1/1
  [mdqo] -> Inverse Park Transform1/1
  Park Transform1/1 -> Demux1/1
  [id_ref] -> Current_controller/1(id-ref)
  In Bus Element3/1 -> Current_controller/5(Vd)
  [iq_ref] -> Current_controller/3(iqref)
  [ipvq] -> Current_controller/4(iq)
  In Bus Element6/1 -> Park Transform1/2
  In Bus Element7/1 -> Inverse Park Transform1/2
  [ipvd] -> Current_controller/2(ipvd)
  In Bus Element5/1 -> Park Transform1/1
  In Bus Element1/1 -> DC voltage controller & current reference/2(Vmag)
  In Bus Element4/1 -> DC voltage controller & current reference/6(LVRT.iq)
  In Bus Element17/1 -> DC voltage controller & current reference/3(P_pv)
  In Bus Element18/1 -> DC voltage controller & current reference/4(PV_Mpp_vdc)
  In Bus Element19/1 -> DC voltage controller & current reference/5(PV_vdc)
  DC voltage controller & current reference/1(iq_ref) -> [iq_ref]
  DC voltage controller & current reference/2(id_ref) -> [id_ref]
  Q_ref/1 -> DC voltage controller & current reference/1(Q_ref)

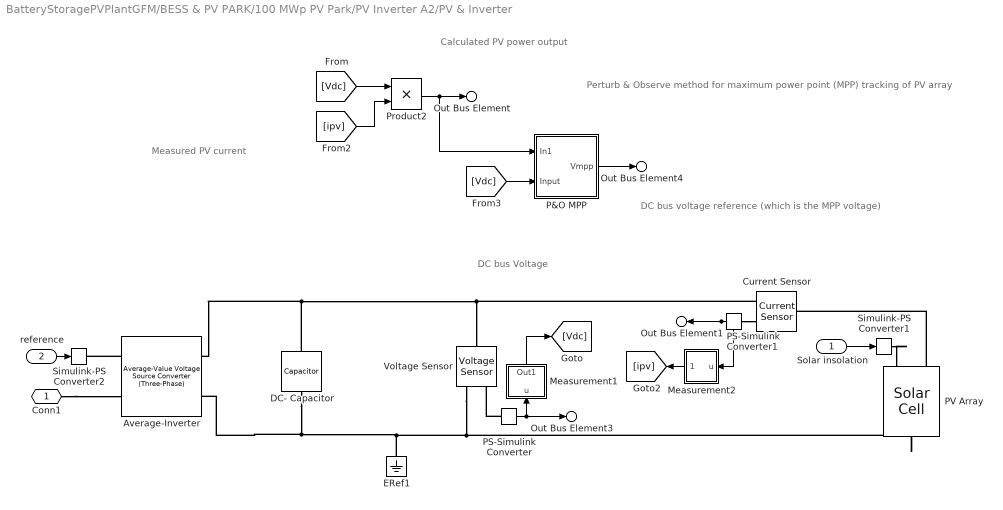
== system BatteryStoragePVPlantGFM/BESS & PV PARK/100 MWp PV Park/PV Inverter A2/PV & Inverter ==
  note: DC bus Voltage
  note: DC bus voltage reference (which is the MPP voltage)
  note: Perturb & Observe method for maximum power point (MPP) tracking of PV array
  note: Measured PV current
  note: Calculated PV power output
  Solar insolation : Inport
  reference : Inport  Port=2
  Average-Inverter : ee_lib/Semiconductors & Converters/Converters/Average-Value Voltage Source Converter (Three-Phase)  port_option=ee.enum.threePhasePort.composite  frequency_option=ee.enum.converters.frequency.variable  FRated=60 Hz  losses_parameterization=ee.enum.converters.losses.fixed  Pfixed=1 W  ks=0.01  kc1=1.7 V  kc2=0.01 Ohm  Ploss_vect=[100, 800, 1870, 3250, 4900] W  Irms_vect=[10, 100, 200, 300, 400] A  Vdc_nom=300 V  thermal_mass=30000 J/K  temperature_specify=off  temperature_priority=High  temperature=298.15 K  temperature_nominal_specify=off  temperature_nominal_unit=K  temperature_nominal_value=1
      settings: InternalSimscapePortConfiguration="{\"Bottom\":[],\"Left\":[{\"id\":\"ModWave\",\"label\":\"ModWave\",\"type\":\"input\"},{\"id\":\"N\",\"label\":\"~\",\"type\":\"foundation.electrical.three_phase\"}],\"Right\":[{\"id\":\"p\",\"label\":\"+\",\"type\":\"foundation.electrical.electrical\"},{\"id\":\"n\",\"label\":\"-\",\"type\":\"foundation.electrical.electrical\"}],\"Top\":[]}"
  Current Sensor : fl_lib/Electrical/Electrical Sensors/Current Sensor
  DC- Capacitor : fl_lib/Electrical/Electrical Elements/Capacitor  c=PVInverter.C F  r=1e-6 Ohm  g=0 1/Ohm  i_specify=off  i_priority=None  i=0 A  i_nominal_specify=off  i_nominal_unit=A  i_nominal_value=1  v_specify=off  v_priority=None  v=6560*.5 V  v_nominal_specify=off  v_nominal_unit=V  v_nominal_value=1  vc_specify=on  vc_priority=None  vc=PVInverter.Vdc V  vc_nominal_specify=off  vc_nominal_unit=V  vc_nominal_value=1
  ERef1 : fl_lib/Electrical/Electrical Elements/Electrical Reference
  Measurement1 : Subsystem
  Measurement2 : Subsystem
  P&O MPP : Subsystem
  PS-Simulink Converter : nesl_utility/PS-Simulink Converter  PhysicalDomain=network_engine_domain  SubClassName=ps_output  LeftPortType=input  RightPortType=output  PseudoPeriodic=off  Frequencies=[]  VectorFormat=inherit  Unit=inherit  AffineConversion=off
  PS-Simulink Converter1 : nesl_utility/PS-Simulink Converter  PhysicalDomain=network_engine_domain  SubClassName=ps_output  LeftPortType=input  RightPortType=output  PseudoPeriodic=off  Frequencies=[]  VectorFormat=inherit  Unit=inherit  AffineConversion=off
  PV Array : ee_lib/Sources/Solar Cell  prm=3  Isc=3.8 A  Voc=0.586 V  Is=SolarCell.diode_saturation_current A  Is2=0 A  Iph=SolarCell.solar_generated_current_AM A  Ir0=1000 W/m^2  ec=SolarCell.quality_factor_i  N2=SolarCell.quality_factor_j  Rs=SolarCell.series_resistance Ohm  Rp=SolarCell.parallel_resistance Ohm  N_series=Panel.n_series_cell_panel*Array.n_series_panels_per_string  N_parallel=Panel.n_parallel_strings_panel*Array.n_parallel_strings  TIPH1=SolarCell.temp_cofficient 1/K  EG=SolarCell.Eg eV  TXIS1=SolarCell.temperature_exponent_Is1  TXIS2=SolarCell.temperature_exponent_Is2  TRS1=SolarCell.temperature_exponent_Rs  TRP1=SolarCell.temperature_exponent_Rp  Tmeas=SolarCell.measurement_temperature degC  TFIXED=SolarCell.device_temperature degC  thermal_mass=100 J/K  initial_temperature=25 degC
  Product2 : Product
  Simulink-PS Converter1 : nesl_utility/Simulink-PS Converter  PhysicalDomain=network_engine_domain  SubClassName=ps_input  LeftPortType=input  RightPortType=output  PseudoPeriodic=off  Frequencies=[]  NoiseDistribution=none  NoiseParameters=[]  Unit=1  AffineConversion=off  FilteringAndDerivatives=provide  SimscapeFilterOrder=1  InputFilterTimeConstant=0.001  UdotUserProvided=0
  Simulink-PS Converter2 : nesl_utility/Simulink-PS Converter  PhysicalDomain=network_engine_domain  SubClassName=ps_input  LeftPortType=input  RightPortType=output  PseudoPeriodic=off  Frequencies=[]  NoiseDistribution=none  NoiseParameters=[]  Unit=1  AffineConversion=off  FilteringAndDerivatives=provide  SimscapeFilterOrder=1  InputFilterTimeConstant=0.001  UdotUserProvided=0
  Voltage Sensor : fl_lib/Electrical/Electrical Sensors/Voltage Sensor
  Conn1 : PMIOPort  Side=Right
  Out Bus Element4 : Outport  PortName=PV_plant1  Element=Vdc_ref
  Out Bus Element : Outport  PortName=PV_plant1  Element=Pref1
  Out Bus Element3 : Outport  PortName=PV_plant1  Element=Vdc_measured
  Out Bus Element1 : Outport  PortName=PV_plant1  Element=ipv
  wires:
  PS-Simulink Converter1/1 -> Measurement2/1(u), Out Bus Element1/1
  Solar insolation/1 -> Simulink-PS Converter1/1
  [ipv] -> Product2/2
  PS-Simulink Converter/1 -> Measurement1/1(u), Out Bus Element3/1
  [Vdc] -> Product2/1
  reference/1 -> Simulink-PS Converter2/1
  Product2/1 -> P&O MPP/1(In1), Out Bus Element/1
  P&O MPP/1(Vmpp) -> Out Bus Element4/1
  [Vdc] -> P&O MPP/2(Input)
  Measurement1/1(Out1) -> [Vdc]
  Measurement2/1(Out1) -> [ipv]
  connections:
  PS-Simulink Converter/LConn1 -- Voltage Sensor/RConn1
  DC- Capacitor/LConn1 -- Current Sensor/RConn2 -- Voltage Sensor/LConn1 -- Average-Inverter/RConn1
  Voltage Sensor/RConn2 -- DC- Capacitor/RConn1 -- Average-Inverter/RConn2 -- ERef1/LConn1 -- PV Array/RConn1
  Average-Inverter/LConn1 -- Simulink-PS Converter2/RConn1
  PV Array/LConn2 -- Current Sensor/LConn1
  Conn1/RConn1 -- Average-Inverter/LConn2
  PS-Simulink Converter1/LConn1 -- Current Sensor/RConn1
  Simulink-PS Converter1/RConn1 -- PV Array/LConn1

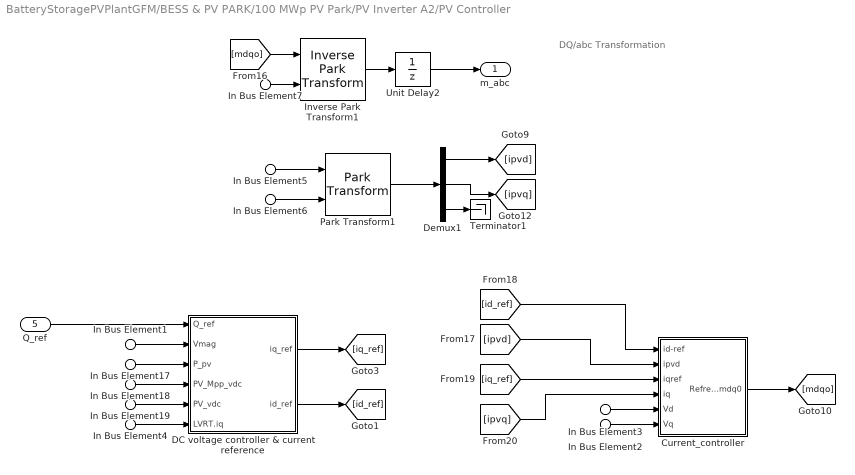
== system BatteryStoragePVPlantGFM/BESS & PV PARK/100 MWp PV Park/PV Inverter A2/PV Controller ==
  note: DQ/abc Transformation
  In Bus Element17 : Inport  PortName=PV_plant1  Element=Pref1
  In Bus Element18 : Inport  PortName=PV_plant1  Element=Vdc_measured
  In Bus Element19 : Inport  PortName=PV_plant1  Element=Vdc_ref
  In Bus Element5 : Inport  Port=2  PortName=ipv1  Element=1
  In Bus Element4 : Inport  Port=3  PortName=LVRT
  In Bus Element3 : Inport  Port=4  PortName=Vbus  Element=Vd
  In Bus Element1 : Inport  Port=4  PortName=Vbus  Element=Vd
  In Bus Element2 : Inport  Port=4  PortName=Vbus  Element=Vq
  In Bus Element6 : Inport  Port=4  PortName=Vbus  Element=Theta
  In Bus Element7 : Inport  Port=4  PortName=Vbus  Element=Theta
  Q_ref : Inport  Port=5
  Current_controller : Subsystem
  DC voltage controller & current reference : Subsystem
  Demux1 : Demux  Outputs=3
  Inverse Park Transform1 : eeTransforms/Inverse Park Transform  AxisAlignment=Q-axis  PowerInvariant=off
  Park Transform1 : eeTransforms/Park Transform  AxisAlignment=Q-axis  PowerInvariant=off
  Terminator1 : Terminator
  Unit Delay2 : UnitDelay  SampleTime=Ts  HasFrameUpgradeWarning=on
  m_abc : Outport
  wires:
  In Bus Element2/1 -> Current_controller/6(Vq)
  Current_controller/1(Refrence_mdq0) -> [mdqo]
  Inverse Park Transform1/1 -> Unit Delay2/1
  Demux1/2 -> [ipvq]
  Unit Delay2/1 -> m_abc/1
  Demux1/1 -> [ipvd]
  Demux1/3 -> Terminator1/1
  [mdqo] -> Inverse Park Transform1/1
  Park Transform1/1 -> Demux1/1
  [id_ref] -> Current_controller/1(id-ref)
  In Bus Element3/1 -> Current_controller/5(Vd)
  [iq_ref] -> Current_controller/3(iqref)
  [ipvq] -> Current_controller/4(iq)
  In Bus Element6/1 -> Park Transform1/2
  In Bus Element7/1 -> Inverse Park Transform1/2
  [ipvd] -> Current_controller/2(ipvd)
  In Bus Element5/1 -> Park Transform1/1
  In Bus Element1/1 -> DC voltage controller & current reference/2(Vmag)
  In Bus Element4/1 -> DC voltage controller & current reference/6(LVRT.iq)
  In Bus Element17/1 -> DC voltage controller & current reference/3(P_pv)
  In Bus Element18/1 -> DC voltage controller & current reference/4(PV_Mpp_vdc)
  In Bus Element19/1 -> DC voltage controller & current reference/5(PV_vdc)
  DC voltage controller & current reference/1(iq_ref) -> [iq_ref]
  DC voltage controller & current reference/2(id_ref) -> [id_ref]
  Q_ref/1 -> DC voltage controller & current reference/1(Q_ref)

== system BatteryStoragePVPlantGFM/BESS & PV PARK/60 MWhr Battery Energy Storage/Variant Subsystem/Grid Following Support ==
  Vbus : Inport
  LVRT : Inport  Port=2
  Battery Inverter : Subsystem
  Current and Voltage Sensor (Three-Phase)5 : ee_lib/Sensors & Transducers/Current and Voltage Sensor (Three-Phase)  vMeasurementType=ee.enum.vmeasurement.lg  outputUnit=ee.enum.unit.pu  SRated=Base.MVA_base_new A*V  VRated=Base.KV_base_new V  I_specify=off  I_priority=None  I=[0, 0, 0] A  I_nominal_specify=off  I_nominal_unit=A  I_nominal_value=1  V_specify=off  V_priority=None  V=[0, 0, 0] V  V_nominal_specify=off  V_nominal_unit=V  V_nominal_value=1
      settings: InternalSimscapePortConfiguration="{\"Bottom\":[],\"Left\":[{\"id\":\"N1\",\"label\":\"~1\",\"type\":\"foundation.electrical.three_phase\"}],\"Right\":[{\"id\":\"V_output\",\"label\":\"V\",\"type\":\"output\"},{\"id\":\"I_output\",\"label\":\"I\",\"type\":\"output\"},{\"id\":\"N2\",\"label\":\"~2\",\"type\":\"foundation.electrical.three_phase\"}],\"Top\":[]}"
  L Filter : ee_lib/Passive/RLC Assemblies/RLC (Three-Phase)  component_structure=ee.enum.rlc.structure.L  R=1e-3 Ohm  L=PVInverter.L H  C=1e-6 F  R_parasitic=0 Ohm  G_parasitic=0 1/Ohm  IL_specify=off  IL_priority=High  IL=[0, 0, 0] A  IL_nominal_specify=off  IL_nominal_unit=A  IL_nominal_value=1  VC_specify=off  VC_priority=High  VC=[0, 0, 0] V  VC_nominal_specify=off  VC_nominal_unit=V  VC_nominal_value=1
      settings: InternalSimscapePortConfiguration="{\"Bottom\":[],\"Left\":[{\"id\":\"N1\",\"label\":\"~1\",\"type\":\"foundation.electrical.three_phase\"}],\"Right\":[{\"id\":\"N2\",\"label\":\"~2\",\"type\":\"foundation.electrical.three_phase\"}],\"Top\":[]}"
  Measurement5 : Subsystem
  PS-Simulink Converter10 : nesl_utility/PS-Simulink Converter  PhysicalDomain=network_engine_domain  SubClassName=ps_output  LeftPortType=input  RightPortType=output  PseudoPeriodic=off  Frequencies=[]  VectorFormat=inherit  Unit=inherit  AffineConversion=off
  PS-Simulink Converter9 : nesl_utility/PS-Simulink Converter  PhysicalDomain=network_engine_domain  SubClassName=ps_output  LeftPortType=input  RightPortType=output  PseudoPeriodic=off  Frequencies=[]  VectorFormat=inherit  Unit=inherit  AffineConversion=off
  GFL1 : PMIOPort  Side=Left
  Bat : Outport
  wires:
  Measurement5/1(ipv1) -> Battery Inverter/2(ipv2)
  Vbus/1 -> Battery Inverter/1(Vbus)
  PS-Simulink Converter9/1 -> Measurement5/2(u)
  LVRT/1 -> Battery Inverter/3(LVRT_iq)
  PS-Simulink Converter10/1 -> Measurement5/1(In1)
  Measurement5/2(Bat) -> Bat/1
  connections:
  PS-Simulink Converter9/LConn1 -- Current and Voltage Sensor (Three-Phase)5/RConn2
  L Filter/LConn1 -- Battery Inverter/RConn1
  GFL1/RConn1 -- Current and Voltage Sensor (Three-Phase)5/RConn3
  Current and Voltage Sensor (Three-Phase)5/LConn1 -- L Filter/RConn1
  Current and Voltage Sensor (Three-Phase)5/RConn1 -- PS-Simulink Converter10/LConn1

== system BatteryStoragePVPlantGFM/BESS & PV PARK/60 MWhr Battery Energy Storage/Variant Subsystem/Grid Forming VSM ==
  Battery Inverter B1 : Subsystem
  Filter & Sensor : Subsystem
  GFL1 : PMIOPort  Side=Left
  Bat : Outport
  wires:
  Filter & Sensor/1(Bat) -> Bat/1, Battery Inverter B1/1(Bat)
  connections:
  GFL1/RConn1 -- Filter & Sensor/RConn1
  Filter & Sensor/LConn1 -- Battery Inverter B1/RConn1

== system BatteryStoragePVPlantGFM/BESS & PV PARK/PV Plant Controller /Voltage VAR Control & LVRT, FRT/Frequency RideThrough ==
  f : Inport
  Avoid Operation : Subsystem
  Discrete-Time Integrator1 : DiscreteIntegrator  ExternalReset=either  SampleTime=Ts  ICPrevOutput=DiscIntNeverNeededParam  ICPrevScaledInput=DiscIntNeverNeededParam
  Duration of f<fth : Lookup_n-D  NumberOfTableDimensions=1  BreakpointsForDimension1=(1+[-0.021,-0.02,0.02,0.021])*Grid.frequency  Table=[1,0,0,1]  InterpMethod=Flat  InternalRulePriority=Speed  RndMeth=Simplest
  Frequency vs Trip time : Lookup_n-D  NumberOfTableDimensions=1  BreakpointsForDimension1=fRT.frequency_x  Table=fRT.time_y  InterpMethod=Flat  InternalRulePriority=Speed  RndMeth=Simplest
  GreaterThan : RelationalOperator  Operator=>  OutDataTypeStr=boolean  RndMeth=Simplest  InputSameDT=off
  Trip  Signal : Outport
  wires:
  Discrete-Time Integrator1/1 -> GreaterThan/1
  Frequency vs Trip time/1 -> GreaterThan/2
  GreaterThan/1 -> Trip  Signal/1
  Duration of f<fth/1 -> Discrete-Time Integrator1/2, Discrete-Time Integrator1/1
  Avoid Operation/1(f) -> Duration of f<fth/1, Frequency vs Trip time/1
  f/1 -> Avoid Operation/1(f_in)

== system BatteryStoragePVPlantGFM/BESS & PV PARK/PV Plant Controller /Voltage VAR Control & LVRT, FRT/LVRT Characterstics ==
  Vmag : Inport
  Discrete-Time Integrator1 : DiscreteIntegrator  ExternalReset=either  SampleTime=Ts  ICPrevOutput=DiscIntNeverNeededParam  ICPrevScaledInput=DiscIntNeverNeededParam
  Duration of Vmag<Vth : Lookup_n-D  NumberOfTableDimensions=1  BreakpointsForDimension1=[0,.9,0.91,1.2]  Table=[1,1,0,0]  InterpMethod=Flat  InternalRulePriority=Speed  RndMeth=Simplest
  Gain1 : Gain  Gain=-1
  GreaterThan : RelationalOperator  Operator=>  OutDataTypeStr=boolean  RndMeth=Simplest  InputSameDT=off
  Saturation2 : Saturate  UpperLimit=1  LowerLimit=-1
  Vmag vs Trip time : Lookup_n-D  NumberOfTableDimensions=1  BreakpointsForDimension1=LVRT.voltage_x  Table=LVRT.time_y  InterpMethod=Flat  InternalRulePriority=Speed  RndMeth=Simplest
  Vmag vs iq : Lookup_n-D  NumberOfTableDimensions=1  BreakpointsForDimension1=LVRT.volatge_iq_x  Table=LVRT.iq_y  InternalRulePriority=Speed  RndMeth=Simplest
  Trip Signal : Outport
  iq : Outport  Port=2
  wires:
  Duration of Vmag<Vth/1 -> Discrete-Time Integrator1/2, Discrete-Time Integrator1/1
  GreaterThan/1 -> Trip Signal/1
  Discrete-Time Integrator1/1 -> GreaterThan/1
  Vmag vs Trip time/1 -> GreaterThan/2
  Vmag vs iq/1 -> Saturation2/1
  Gain1/1 -> iq/1
  Saturation2/1 -> Gain1/1
  Vmag/1 -> Vmag vs iq/1, Vmag vs Trip time/1, Duration of Vmag<Vth/1
